simulink model "CSE_BDA_SIMULINK_NO2_CASTOR_FAJANILAN"  (R2024a)
settings: Solver=VariableStepAuto  StartTime=0.0  StopTime=20  RelTol=1e-3
values from neighbouring files (symbols this model uses):
  G1_den = [1 0 0]    [CSE_BDA_NO2_CASTOR_FAJANILAN.m]
  G1_num = [0 0 1]    [CSE_BDA_NO2_CASTOR_FAJANILAN.m]
  G1G2_den = conv(G1_den,G2_den)    [CSE_BDA_NO2_CASTOR_FAJANILAN.m]
  G1G2_num = conv(G1_num,G2_num)    [CSE_BDA_NO2_CASTOR_FAJANILAN.m]
  G1G2G3G4H1H2H3_den = G1G2G3G4H1H2H3_multi + [0 0 0 0 0 0 1 -3 2]    [CSE_BDA_NO2_CASTOR_FAJANILAN.m]
  G1G2G3G4H1H2H3_num = conv(H1_num,G1G2G3G4H2H1_num)    [CSE_BDA_NO2_CASTOR_FAJANILAN.m]
  G1G2G3G4H2H1_den = conv(G2G3G4H2H3_den,G1_den)    [CSE_BDA_NO2_CASTOR_FAJANILAN.m]
  G1G2G3G4H2H1_num = [1 -3 2]    [CSE_BDA_NO2_CASTOR_FAJANILAN.m]
  G2_den = [1 1]    [CSE_BDA_NO2_CASTOR_FAJANILAN.m]
  G2_num = [0 0 1]    [CSE_BDA_NO2_CASTOR_FAJANILAN.m]
  G2G3G4H2H3_den = G2G3G4H2H3_multi + [0 0 0 1 0 -1]    [CSE_BDA_NO2_CASTOR_FAJANILAN.m]
  G2G3G4H2H3_num = conv(G3G2H2_num,H3_den)    [CSE_BDA_NO2_CASTOR_FAJANILAN.m]
  G3_den = [1 0]    [CSE_BDA_NO2_CASTOR_FAJANILAN.m]
  G3_num = [0 1]    [CSE_BDA_NO2_CASTOR_FAJANILAN.m]
  G3G2H2_den = G3G2H2_den_multi + G3G2H2_den_add    [CSE_BDA_NO2_CASTOR_FAJANILAN.m]
  G3G2H2_num = conv(G2H2_den,G3_num)    [CSE_BDA_NO2_CASTOR_FAJANILAN.m]
  G4_den = [2 0]    [CSE_BDA_NO2_CASTOR_FAJANILAN.m]
  G4_num = [1]    [CSE_BDA_NO2_CASTOR_FAJANILAN.m]
  H1_den = [1 0]    [CSE_BDA_NO2_CASTOR_FAJANILAN.m]
  H1_num = [0 1]    [CSE_BDA_NO2_CASTOR_FAJANILAN.m]
  H2_den = [1 -1]    [CSE_BDA_NO2_CASTOR_FAJANILAN.m]
  H2_num = [0 1]    [CSE_BDA_NO2_CASTOR_FAJANILAN.m]
  H3_den = [1 -2]    [CSE_BDA_NO2_CASTOR_FAJANILAN.m]
  H3_num = [0 1]    [CSE_BDA_NO2_CASTOR_FAJANILAN.m]
settings Model: Creator=User  LastModifiedBy=HP
settings SolverCC: AlgebraicLoopSolver=TrustRegion
settings DebuggingCC: UnconnectedInputMsg=warning  UnconnectedOutputMsg=warning  UnconnectedLineMsg=warning
settings ModelReferenceCC: EnableRefExpFcnMdlSchedulingChecks=on
settings SFSimCC: CustomCodeUndefinedFunction=UseInterfaceOnly
settings RTWCC: GPUComputeCapability=3.5

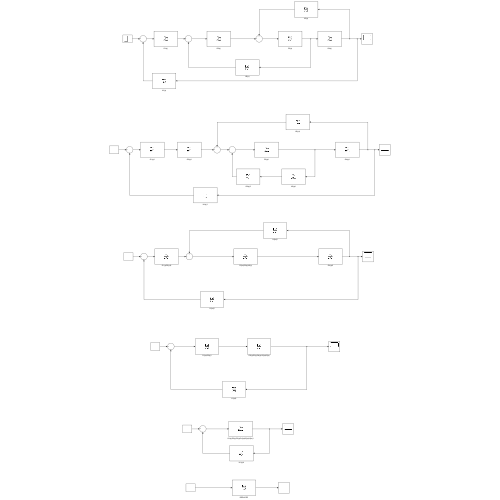
[thumbnail: Simulink's stored preview of the top-level diagram]
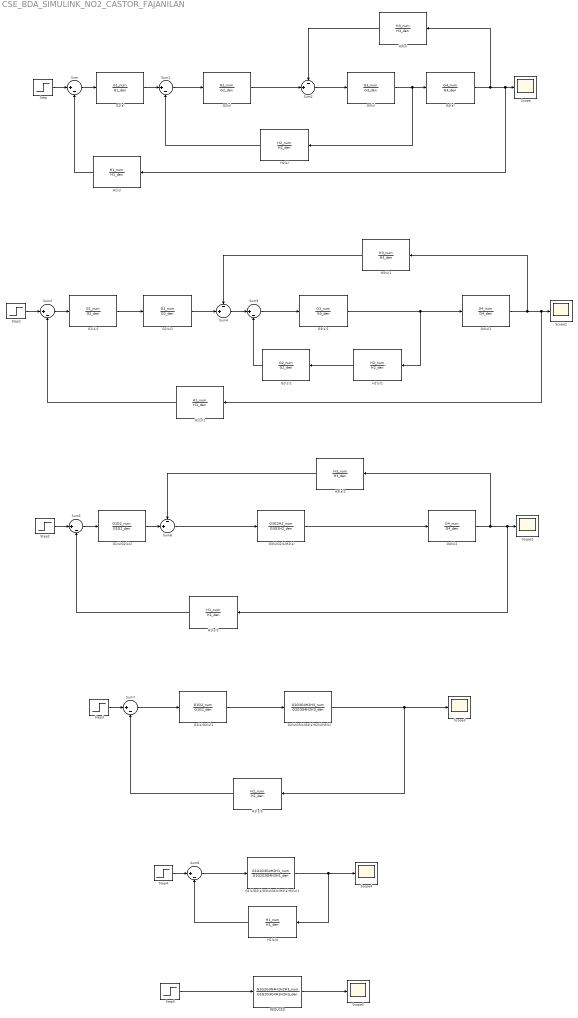
== system CSE_BDA_SIMULINK_NO2_CASTOR_FAJANILAN ==
  G1(s) : TransferFcn  Numerator=G1_num  Denominator=G1_den
  G1(s)1 : TransferFcn  Numerator=G1_num  Denominator=G1_den
  G1(s)G2(s)1 : TransferFcn  Numerator=G1G2_num  Denominator=G1G2_den
  G1(s)G2(s)2 : TransferFcn  Numerator=G1G2_num  Denominator=G1G2_den
  G1(s)G2(s)G3(s)G4(s)H2(s)H3(s)1 : TransferFcn  Numerator=G1G2G3G4H2H1_num  Denominator=G1G2G3G4H2H1_den
  G2(s) : TransferFcn  Numerator=G2_num  Denominator=G2_den
  G2(s)1 : TransferFcn  Numerator=G2_num  Denominator=G2_den
  G2(s)2 : TransferFcn  Numerator=G2_num  Denominator=G2_den
  G2(s)G3(s)G4(s)H2(s)H3(s) : TransferFcn  Numerator=G2G3G4H2H3_num  Denominator=G2G3G4H2H3_den
  G3(s) : TransferFcn  Numerator=G3_num  Denominator=G3_den
  G3(s)1 : TransferFcn  Numerator=G3_num  Denominator=G3_den
  G3(s)G2(s)H2(s) : TransferFcn  Numerator=G3G2H2_num  Denominator=G3G2H2_den
  G4(s) : TransferFcn  Numerator=G4_num  Denominator=G4_den
  G4(s)1 : TransferFcn  Numerator=G4_num  Denominator=G4_den
  G4(s)2 : TransferFcn  Numerator=G4_num  Denominator=G4_den
  H1(s){,1..4} (5 alike) : TransferFcn  Numerator=H1_num  Denominator=H1_den
  H2(s) : TransferFcn  Numerator=H2_num  Denominator=H2_den
  H2(s)1 : TransferFcn  Numerator=H2_num  Denominator=H2_den
  H3(s) : TransferFcn  Numerator=H3_num  Denominator=H3_den
  H3(s)1 : TransferFcn  Numerator=H3_num  Denominator=H3_den
  H3(s)2 : TransferFcn  Numerator=H3_num  Denominator=H3_den
  REDUCED : TransferFcn  Numerator=G1G2G3G4H1H2H3_num  Denominator=G1G2G3G4H1H2H3_den
  Scope{,1..5} (6 alike) : Scope
  Step{,1..5} (6 alike) : Step  SampleTime=0
  Sum{,1,3,5,7..9} (7 alike) : Sum  Inputs=|+-
  Sum2 : Sum  Inputs=-+|
  Sum4 : Sum  Inputs=-+|
  Sum6 : Sum  Inputs=-+|
  wires:
  Step/1 -> Sum/1
  Sum/1 -> G1(s)/1
  G1(s)/1 -> Sum1/1
  H1(s)/1 -> Sum/2
  Sum1/1 -> G2(s)/1
  G2(s)/1 -> Sum2/2
  Sum2/1 -> G3(s)/1
  H3(s)/1 -> Sum2/1
  G3(s)/1 -> H2(s)/1, G4(s)/1
  G4(s)/1 -> H1(s)/1, Scope/1, H3(s)/1
  H2(s)/1 -> Sum1/2
  G4(s)1/1 -> H3(s)1/1, H1(s)1/1, Scope1/1
  H1(s)1/1 -> Sum3/2
  G3(s)1/1 -> G4(s)1/1, H2(s)1/1
  Step1/1 -> Sum3/1
  Sum3/1 -> G1(s)1/1
  Sum6/1 -> G3(s)G2(s)H2(s)/1
  Sum5/1 -> G1(s)G2(s)2/1
  Step2/1 -> Sum5/1
  H1(s)2/1 -> Sum5/2
  G3(s)G2(s)H2(s)/1 -> G4(s)2/1
  Step3/1 -> Sum7/1
  H1(s)3/1 -> Sum7/2
  G1(s)G2(s)1/1 -> G2(s)G3(s)G4(s)H2(s)H3(s)/1
  Sum7/1 -> G1(s)G2(s)1/1
  G2(s)G3(s)G4(s)H2(s)H3(s)/1 -> Scope3/1, H1(s)3/1
  Step4/1 -> Sum8/1
  H1(s)4/1 -> Sum8/2
  Sum8/1 -> G1(s)G2(s)G3(s)G4(s)H2(s)H3(s)1/1
  G1(s)G2(s)G3(s)G4(s)H2(s)H3(s)1/1 -> H1(s)4/1, Scope4/1
  REDUCED/1 -> Scope5/1
  Step5/1 -> REDUCED/1
  H2(s)1/1 -> G2(s)2/1
  H3(s)1/1 -> Sum4/1
  G1(s)1/1 -> G2(s)1/1
  G2(s)1/1 -> Sum4/2
  Sum4/1 -> Sum9/1
  Sum9/1 -> G3(s)1/1
  G2(s)2/1 -> Sum9/2
  G1(s)G2(s)2/1 -> Sum6/2
  H3(s)2/1 -> Sum6/1
  G4(s)2/1 -> H3(s)2/1, H1(s)2/1, Scope2/1
